simulink model "nl_pla_filter"  (R2020b)
settings: Solver=FixedStepDiscrete  StartTime=0.0  StopTime=stopTime  FixedStep=2.0833333333333333e-05  RelTol=1e-3
values from neighbouring files (symbols this model uses):
  cf_factor = min(cfsat, 10^(cfslope*cf/1e3 + cfconst)) * 2.0    [NLBeforePLA.m]
  multFac = max(2.95*max(1.0,1.5-spont/100), 4.3-0.2*cf/1e3)    [NLBeforePLA.m]
undefined symbols (not defined in the file or in its folder): spont
libraries: simulink x1
settings Model: Creator=Ross  LastModifiedBy=conno
settings DataIOCC: SaveOutput=off  SaveTime=off  ReturnWorkspaceOutputs=off
settings OptimizationCC: BlockReduction=off  ConditionallyExecuteInputs=off  DefaultParameterBehavior=Inlined
settings DebuggingCC: ReadBeforeWriteMsg=DisableAll  WriteAfterWriteMsg=DisableAll  WriteAfterReadMsg=DisableAll  AlgebraicLoopMsg=error  MultiTaskDSMMsg=none  SingleTaskRateTransMsg=error  PregeneratedLibrarySubsystemCodeDiagnostic=none  ArithmeticOperatorsInVariantConditions=warning
settings HardwareCC: ProdBitPerPointer=32  ProdBitPerSizeT=32  ProdBitPerPtrDiffT=32  ProdLargestAtomicFloat=None  ProdIntDivRoundTo=Undefined  ProdEndianess=Unspecified  ProdWordSize=32  ProdHWDeviceType=ASIC/FPGA->ASIC/FPGA  TargetBitPerPointer=64  TargetBitPerSizeT=64  TargetBitPerPtrDiffT=64  TargetLongLongMode=on  TargetIntDivRoundTo=Zero  TargetEndianess=LittleEndian  TargetWordSize=64  TargetHWDeviceType=Custom Processor->MATLAB Host Computer  ProdEqTarget=off
settings ModelReferenceCC: UpdateModelReferenceTargets=IfOutOfDate
settings SFSimCC: SFSimEcho=off  SimUseLocalCustomCode=off  CustomCodeUndefinedFunction=UseInterfaceOnly
settings RTWCC: RTWUseLocalCustomCode=off

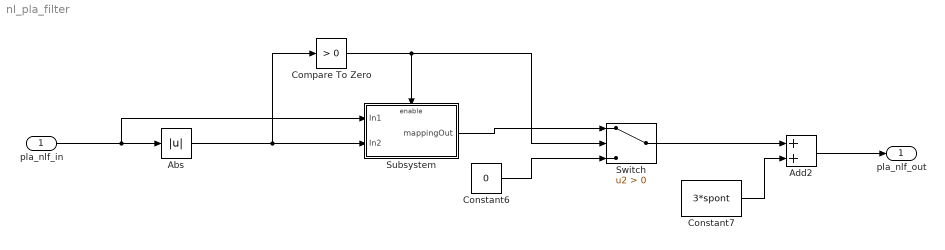
== system nl_pla_filter ==
  pla_nlf_in : Inport  OutDataTypeStr=single  PortDimensions=1  SampleTime=[2.0833333333333333e-05,0]
  Abs : Abs
  Add2 : Sum
  Compare To Zero : simulink/Logic and Bit Operations/Compare To Zero  relop=>  OutDataTypeStr=boolean
  Constant6 : Constant  Value=0  OutDataTypeStr=single  SampleTime=-1
  Constant7 : Constant  Value=3*spont  OutDataTypeStr=single  SampleTime=-1
  Subsystem : Subsystem
  Switch : Switch  Criteria=u2 > Threshold  OutDataTypeStr=single
  pla_nlf_out : Outport  OutDataTypeStr=single  PortDimensions=1  SampleTime=[2.0833333333333333e-05,0]  VectorParamsAs1DForOutWhenUnconnected=off
  wires:
  Compare To Zero/1 -> Subsystem/Enable, Switch/2
  Subsystem/1(mappingOut) -> Switch/1
  Abs/1 -> Compare To Zero/1, Subsystem/2(In2)
  pla_nlf_in/1 -> Subsystem/1(In1), Abs/1
  Add2/1 -> pla_nlf_out/1
  Constant7/1 -> Add2/2
  Switch/1 -> Add2/1
  Constant6/1 -> Switch/3

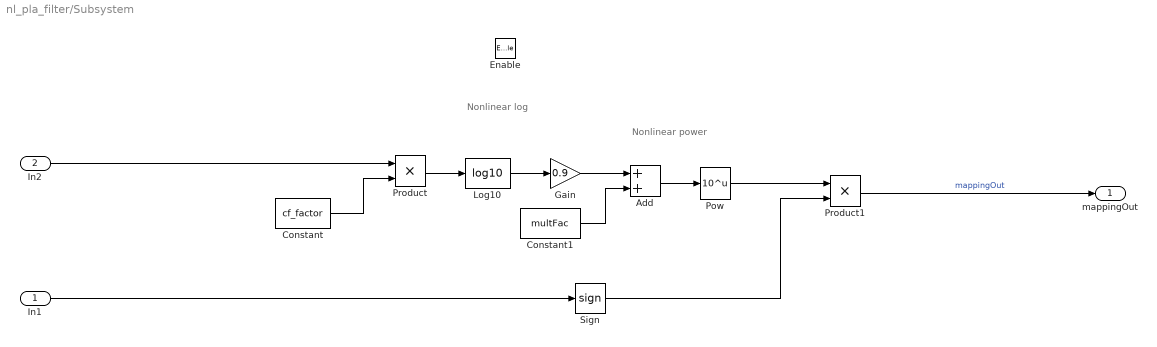
== system nl_pla_filter/Subsystem ==
  note: Nonlinear log
  note: Nonlinear power
  In1 : Inport
  In2 : Inport  Port=2
  Enable : EnablePort
  Add : Sum
  Constant : Constant  Value=cf_factor  OutDataTypeStr=single  SampleTime=-1
  Constant1 : Constant  Value=multFac  OutDataTypeStr=single  SampleTime=-1
  Gain : Gain  Gain=0.9
  Log10 : Math  Operator=log10  SignedPower=on  RndMeth=Zero  SaturateOnIntegerOverflow=on
  Pow : Math  Operator=10^u  SignedPower=on  RndMeth=Zero  SaturateOnIntegerOverflow=on
  Product : Product
  Product1 : Product
  Sign : Signum
  mappingOut : Outport  InitialOutput=[0]
  wires:
  Pow/1 -> Product1/1
  Constant/1 -> Product/2
  Product/1 -> Log10/1
  Log10/1 -> Gain/1
  Gain/1 -> Add/1
  Add/1 -> Pow/1
  Constant1/1 -> Add/2
  In2/1 -> Product/1
  Product1/1 -> mappingOut/1  "mappingOut"
  In1/1 -> Sign/1
  Sign/1 -> Product1/2
